simulink model "ACC_Ver01_CoreControl"  (R2026a)
settings: Solver=FixedStepAuto  StopTime=inf  FixedStep=0.1
settings Model: Creator=Rakshith  LastModifiedBy=Rakshith

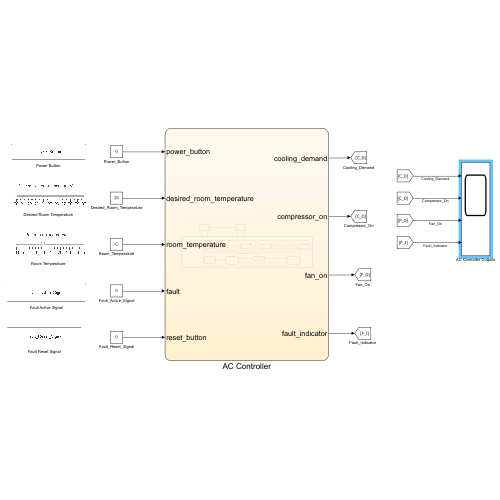
[thumbnail: Simulink's stored preview of the top-level diagram]
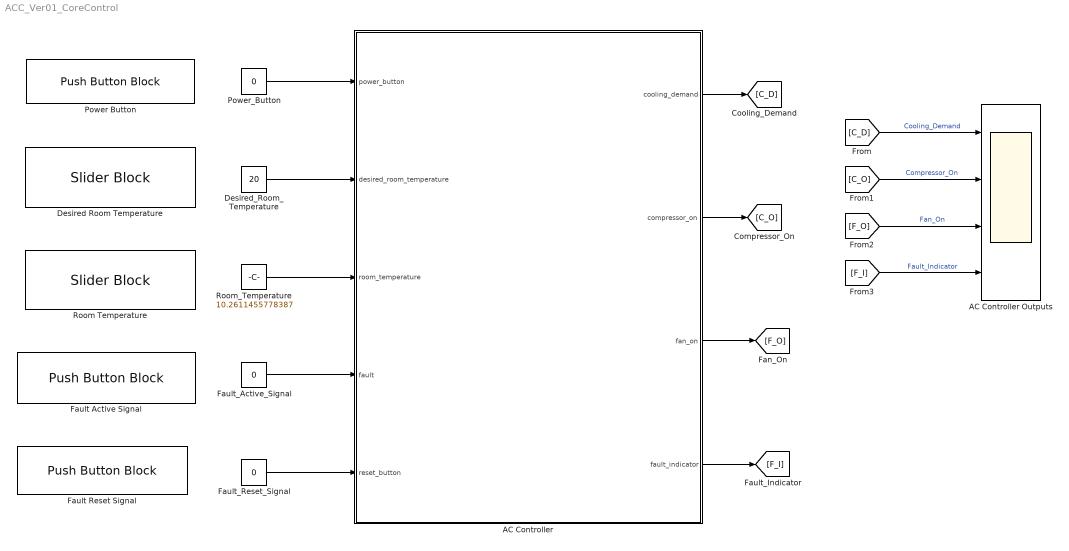
== system ACC_Ver01_CoreControl ==
  AC Controller : Stateflow chart  TreatAsAtomicUnit=on
  AC Controller Outputs : Scope  NumInputPorts=4
      settings: ActiveDisplayYMinimum=-0.12499999999999997  ActiveDisplayYMaximum=1.125
  Desired Room Temperature : SliderBlock  ScaleMin=20  ScaleMax=30
  Desired_Room_Temperature : Constant  Value=20
  Fault Active Signal : PushButtonBlock  ButtonText=Fault_Active_Signal  ButtonType=Latch  IconOnColor=[0.0, 0.39215686274509803, 0.0]  IconOffColor=[0.0, 1.0, 0.0]  OffValue=0.000000
  Fault Reset Signal : PushButtonBlock  ButtonText=Fault_Reset_Signal  ButtonType=Latch  IconOnColor=[0.0, 0.39215686274509803, 0.0]  IconOffColor=[0.0, 1.0, 0.0]  OffValue=0.000000
  Fault_Active_Signal : Constant  Value=0
  Fault_Reset_Signal : Constant  Value=0
  Power Button : PushButtonBlock  ButtonText=Power_Button  ButtonType=Latch  IconOnColor=[0.0, 0.39215686274509803, 0.0]  IconOffColor=[0.0, 1.0, 0.0]  OffValue=0.000000
  Power_Button : Constant  Value=0
  Room Temperature : SliderBlock  ScaleMin=-80  ScaleMax=150
  Room_Temperature : Constant  Value=10.2611455778387
  wires:
  AC Controller/4(fault_indicator) -> [F_I]
  [C_D] -> AC Controller Outputs/1  "Cooling_Demand"
  AC Controller/2(compressor_on) -> [C_O]
  Fault_Reset_Signal/1 -> AC Controller/5(reset_button)
  [F_O] -> AC Controller Outputs/3  "Fan_On"
  AC Controller/3(fan_on) -> [F_O]
  [C_O] -> AC Controller Outputs/2  "Compressor_On"
  Desired_Room_Temperature/1 -> AC Controller/2(desired_room_temperature)
  [F_I] -> AC Controller Outputs/4  "Fault_Indicator"
  Power_Button/1 -> AC Controller/1(power_button)
  Fault_Active_Signal/1 -> AC Controller/4(fault)
  Room_Temperature/1 -> AC Controller/3(room_temperature)
  AC Controller/1(cooling_demand) -> [C_D]

== stateflow chart ACC_Ver01_CoreControl/AC Controller ==
  state Power_Off
    en: compressor_on = 0;
    fan_on = 0;
    cooling_demand = 0;
    fault_indicator = 0;
  state Fault_State
    en: compressor_on = 0;
    fan_on = 0;
    cooling_demand = 0;
    fault_indicator = 1;
  state Power_On
    en: fault_indicator = 0;
    du: set_temperature = desired_room_temperature;
    temperature_error = room_temperature-set_temperature;
    state Cooling_Demand [parallel]
      settings: executionOrder=1
      state Cooling_Demand_Activation
        en: cooling_demand = 1;
      state Cooling_Demand_Deactivation
        en: cooling_demand = 0;
      (default) -> Cooling_Demand_Deactivation
      Cooling_Demand_Deactivation -> Cooling_Demand_Activation : [ temperature_error >= temperature_hysteresis_band ]
      Cooling_Demand_Activation -> Cooling_Demand_Deactivation : [ temperature_error <= -temperature_hysteresis_band ]
    state Compressor_Mechanism [parallel]
      settings: executionOrder=2
      state Compressor_Activation
        en: compressor_on = 1;
      state Compressor_Deactivation
        en: compressor_on = 0;
      (default) -> Compressor_Deactivation
      Compressor_Deactivation -> Compressor_Activation : [ after(compressor_min_off_time, sec) && cooling_demand == 1 ]
      Compressor_Activation -> Compressor_Deactivation : [ cooling_demand == 0 ]
    state Fan_Mechanism [parallel]
      settings: executionOrder=3
      state Fan_Activation
        en: fan_on = 1;
      state Compressor_Off_Check
        en: fan_on = 1;
      state Fan_Deactivation
        en: fan_on = 0;
      state Fan_On_Standby
        en: fan_on = 1;
      Compressor_Off_Check -> Fan_Activation [order 1] : [ compressor_on == 1 ]
      (default) -> Fan_On_Standby
      Fan_Activation -> Compressor_Off_Check : [ compressor_on == 0 ]
      Compressor_Off_Check -> Fan_Deactivation [order 2] : [ after(fan_run_on_time, sec) && compressor_on == 0 ]
      Fan_On_Standby -> Fan_Activation : [ compressor_on == 1 ]
      Fan_Deactivation -> Fan_Activation : [ compressor_on == 1 ]
  (default) -> Power_Off
  Fault_State -> Power_Off [order 2] : [ (reset_button ==1 && fault == 0) && power_button == 0 ]
  Power_On -> Power_Off [order 2] : [ power_button == 0 ]
  Power_Off -> Power_On : [ power_button == 1 ]
  Fault_State -> Power_On [order 1] : [ (reset_button ==1 && fault == 0) && power_button == 1 ]
  Power_On -> Fault_State [order 1] : [ fault == 1 ]
  data: cooling_demand output; compressor_on output; power_button input; compressor_min_off_time local =15; desired_room_temperature input; fan_run_on_time local =2*60; room_temperature input; fault input; reset_button input; temperature_hysteresis_band local =7.5; fan_on output; fault_indicator output; set_temperature local =0; temperature_error local =0
